simulink model "example_model_doc"  (R2016b)
settings: Solver=ode45  StartTime=0.0  StopTime=10  RelTol=1e-3
libraries: carnot x7
settings Model: Creator=goettsche  LastModifiedBy=drhf
settings DataIOCC: LimitDataPoints=on  SaveFormat=Array  SignalLoggingSaveFormat=ModelDataLogs  ReturnWorkspaceOutputs=on
settings OptimizationCC: LifeSpan=inf
settings DebuggingCC: ReadBeforeWriteMsg=DisableAll  WriteAfterWriteMsg=DisableAll  WriteAfterReadMsg=DisableAll  SaveWithParameterizedLinksMsg=none  UnderspecifiedInitializationDetection=Classic  MergeDetectMultiDrivingBlocksExec=none  MultiTaskDSMMsg=none  MultiTaskCondExecSysMsg=none  SFUnexpectedBacktrackingDiag=warning  SFNoUnconditionalDefaultTransitionDiag=warning  SFExecutionAtInitializationDiag=none
settings HardwareCC: ProdBitPerPointer=32  ProdBitPerSizeT=32  ProdBitPerPtrDiffT=32  ProdLargestAtomicFloat=None  ProdIntDivRoundTo=Undefined  ProdEndianess=Unspecified  ProdWordSize=32  ProdHWDeviceType=32-bit Generic  TargetUnknown=on
settings ModelReferenceCC: UpdateModelReferenceTargets=IfOutOfDate  PropagateSignalLabelsOutOfModel=off
settings SFSimCC: SFSimEcho=off
settings GRTTargetCC: TargetLangStandard=C89/C90 (ANSI)  GeneratePreprocessorConditionals=Disable all
settings ConfigComp: CovMetricSettings=dw  CovHtmlReporting=on  CovSaveCumulativeToWorkspaceVar=on  CovSaveSingleToWorkspaceVar=on  CovExternalEMLEnable=off

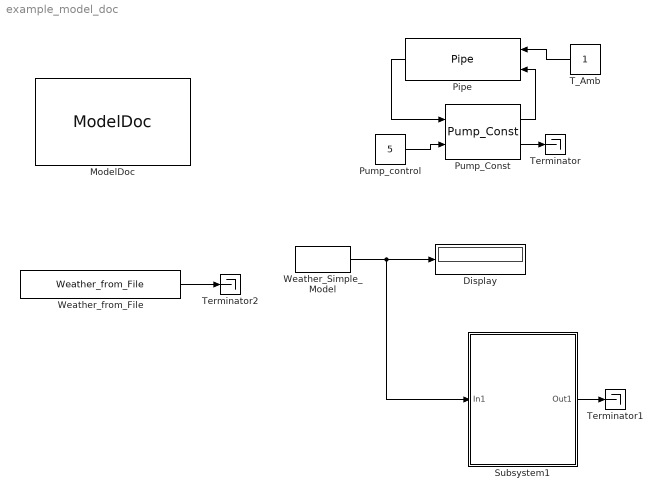
== system example_model_doc ==
  " ModelDoc" : carnot/Toolbox/ ModelDoc  SystemSampleTime=-1
  Display : Display
  Pipe : carnot/Hydraulics/Pipe  dia=0.02  len=10  hgt=5  uloss=100/20/10  cond=0  cwall=1000  t0=20  lin=100/0.2  qua=100/0.2^2  nodes=10
  Pump_Const : carnot/Hydraulics/Pump_Const  mdotmax=1200/3600  dia=0.0157  power=30  p0=3e5  fluid_id=Water  mix=0  UA=3  mcp=4000  tamb=20
  Pump_control : Constant  Value=5
  Subsystem1 : Subsystem  TreatAsAtomicUnit=on
  T_Amb : Constant
  Terminator : Terminator
  Terminator1 : Terminator
  Terminator2 : Terminator
  Weather_Simple_Model : carnot/Weather/Weather_Simple_Model  lat=60  Ibn=900  Idg=100  tamb=5  deltaTsky=-6  rh=50  precip="10e-3/24/3600           % 10 mm in 24 h"  cloud=0.125  p=1013e2  vw=1  wdir=270
  Weather_from_File : carnot/Weather/Weather_from_File  file=DE_TRY2010_04_averageYear  ext=.mat
  wires:
  Weather_Simple_Model/1 -> Subsystem1/1(In1), Display/1
  Pump_control/1 -> Pump_Const/2
  Pump_Const/1 -> Pipe/2
  Pipe/1 -> Pump_Const/1
  T_Amb/1 -> Pipe/1
  Pump_Const/2 -> Terminator/1
  Subsystem1/1(Out1) -> Terminator1/1
  Weather_from_File/1 -> Terminator2/1

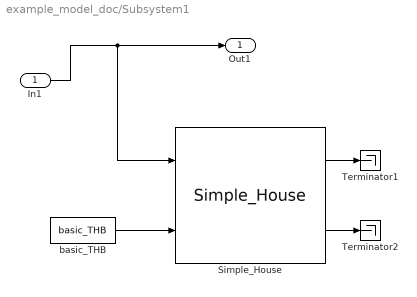
== system example_model_doc/Subsystem1 ==
  In1 : Inport
  Simple_House : carnot/Load/Houses/Simple_House  Ahabit=30  Hroom=2.5  Floorsize=[5 6]  UAwall=0.162*(30)+0.182*((5+6)*2*2.5 -(4+0+0+0))  UAneighbour=0  Uground="0  %0.18 wenn Wert verlangt"  mc="0.5e6*30   % 0.5 MJ/m2/K"  shade=0.75  tini=20  Awin=[4 0 0 0]  AziWin=[0 90 -180 -90]  Uwin="[1    1   1    1]*1.5"  Gwin="[1    1   1    1]*0.7*(1-0.15)"  vent=0.4  rec=0  heatload=2000  dpcoeff=[10 100]  delta_t_nom=50  n_rad=1.1  mass_times_cap=40e6
  Terminator1 : Terminator
  Terminator2 : Terminator
  basic_THB : carnot/Basic/Hydraulics/basic_THB  t=10  mdot=100/3600  p=2e5  ID=1  fluid=1  mix=0  mix2=0  mix3=0  dia=.03  hgt=1
  Out1 : Outport
  wires:
  In1/1 -> Simple_House/1, Out1/1
  basic_THB/1 -> Simple_House/2
  Simple_House/1 -> Terminator1/1
  Simple_House/2 -> Terminator2/1
